simulink library "BSPD"  (R2024a)
settings: Solver=VariableStepAuto  StartTime=0.0  StopTime=10.0  RelTol=1e-3
undefined symbols (not defined in the file): raptor_xcp_function
libraries: Utilities x2, Raptor_lib x2
settings Model: Creator=serga  LastModifiedBy=serga

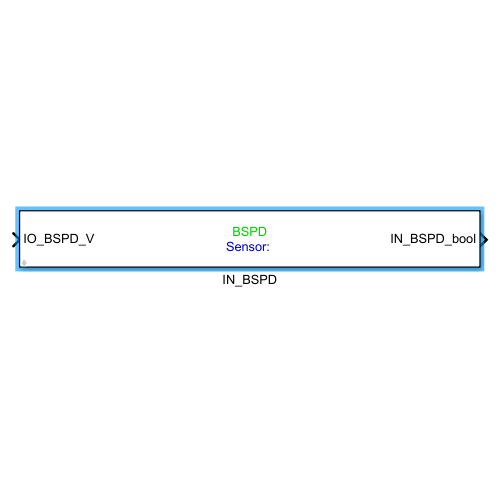
[thumbnail: Simulink's stored preview of the top-level diagram]
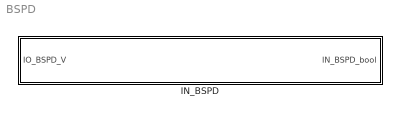
== system BSPD ==
  IN_BSPD : Subsystem  mask{pos=''}
      mask prompts: pos "Position"
      mask Display:
      | color('green')
      | disp('BSPD\n');
      | color('blue')
      | disp(['\nSensor: ' pos]);
      | color('black')
      | port_label('input', 1, ['IO_BSPD' pos '_V']);
      | port_label('output', 1, ['IN_BSPD' pos '_bool']);

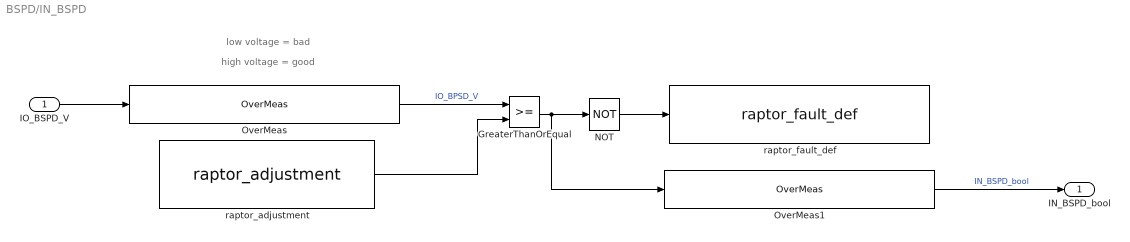
== system BSPD/IN_BSPD ==
  note: high voltage = good
  note: low voltage = bad
  IO_BSPD_V : Inport
  GreaterThanOrEqual : RelationalOperator  OutDataTypeStr=boolean  RndMeth=Simplest  InputSameDT=off
  NOT : Logic  Operator=NOT  AllPortsSameDT=off  OutDataTypeStr=boolean
  OverMeas : Utilities/OverMeas  sigName=['IO_BPSD' pos '_V']  min=0  max=5
  OverMeas1 : Utilities/OverMeas  sigName=['IN_BSPD' pos '_bool']  min=0  max=1
  raptor_adjustment : Raptor_lib/Data Storage/raptor_adjustment  paramName=['IN_BSPD' pos 'HighThresh_V']  nameSource=Parameter  initValue=3  dataType=single  storage=Calibration  calDispType=Number  calEnum={'False', 'True'}  calGain=1.0  calOffset=0.0  calMax=5  calMin=0  calFormat='-1'  calUnit=''  calHelp=''  calAccess=1  calFunction=raptor_xcp_function(gcb)  calDispHeaders=off  calColHeaders={'Col1' 'Col2' 'Col3'}  calRowHeaders={'Row1' 'Row2' 'Row3'}
      settings: SourceProductName=Raptor
  raptor_fault_def : Raptor_lib/Faults/raptor_fault_def  faultName=['IN_BSPD' pos 'Fault']  persist=off  sticky=off  emisRelated=off  singleTrip=off  clearMethod=Standard  xLimit=25  yLimit=50  calEnable=on  addDisable=off  calAccess=1  calFunction='System | FaultManager'
      settings: SourceProductName=Raptor
  IN_BSPD_bool : Outport
  wires:
  OverMeas1/1 -> IN_BSPD_bool/1  "IN_BSPD_bool"
  OverMeas/1 -> GreaterThanOrEqual/1  "IO_BPSD_V"
  IO_BSPD_V/1 -> OverMeas/1
  raptor_adjustment/1 -> GreaterThanOrEqual/2
  NOT/1 -> raptor_fault_def/1
  GreaterThanOrEqual/1 -> OverMeas1/1, NOT/1
